simulink model "gimbal_kinematics_model_mpc_v2_19012020"  (R2018b)
settings: Solver=FixedStepAuto  StartTime=0.0  StopTime=10  FixedStep=0.001  MaxStep=0.001  RelTol=1e-3
libraries: robotcorelib x5, mpclib x1
settings Model: Creator=Paweł Tymiński  LastModifiedBy=Paweł Tymiński

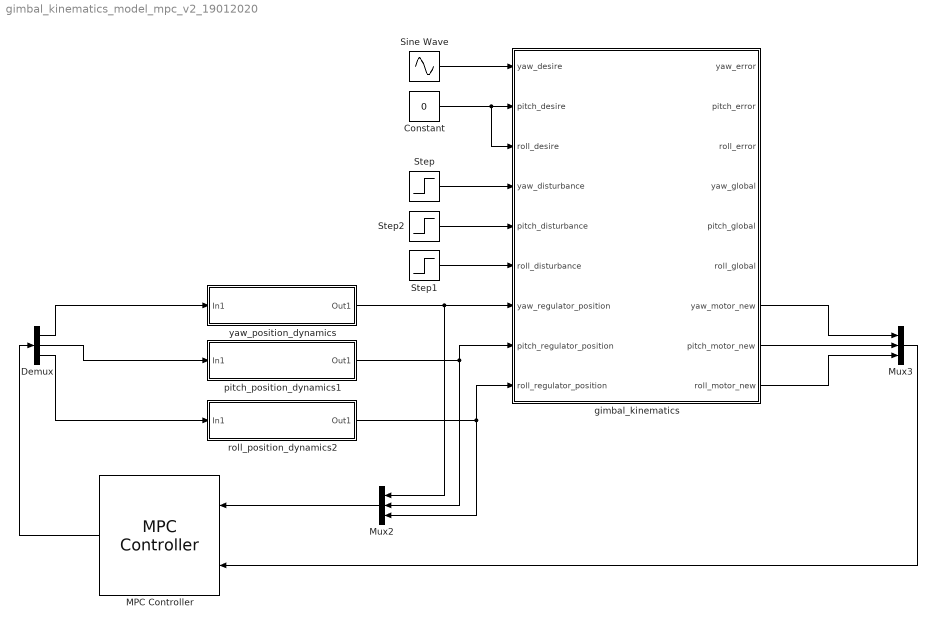
== system gimbal_kinematics_model_mpc_v2_19012020 ==
  Constant : Constant  Value=0
  Demux : Demux  Outputs=3
  MPC Controller : mpclib/MPC Controller  SCDEnableBlockLinearizationSpecification=on  is_multiple=0  enable_value=0  return_u0=off  updateMPCinCallerWorkspace=on  md_inport=off  mv_inport=off  return_cost=off  return_mvseq=off  return_qpstatus=off  return_xseq=off  return_state=off  return_ovseq=off  state_inport=off  umin_inport=off  umax_inport=off  ymin_inport=off  ymax_inport=off  cc_inport=off  ywt_inport=off  uwt_inport=off  duwt_inport=off  rhoeps_inport=off  uref_inport=off  n_ts=0.001  n_p=10  n_mv=3  n_md=0  n_ud=0  n_mo=3  n_uo=0  BlockDataType=double  SampleTimeInherited=off  switch_inport=off
  Mux2 : Mux  Inputs=3
  Mux3 : Mux  Inputs=3
  Sine Wave : Sin  SampleTime=0
  Step : Step  Time=2  After=-0.5  SampleTime=0
  Step1 : Step  Time=2  After=-1  SampleTime=0
  Step2 : Step  Time=5  After=0.5  SampleTime=0
  gimbal_kinematics : Subsystem
  pitch_position_dynamics1 : Subsystem
  roll_position_dynamics2 : Subsystem
  yaw_position_dynamics : Subsystem
  wires:
  pitch_position_dynamics1/1(Out1) -> gimbal_kinematics/8(pitch_regulator_position), Mux2/2
  roll_position_dynamics2/1(Out1) -> gimbal_kinematics/9(roll_regulator_position), Mux2/3
  yaw_position_dynamics/1(Out1) -> Mux2/1, gimbal_kinematics/7(yaw_regulator_position)
  Constant/1 -> gimbal_kinematics/3(roll_desire), gimbal_kinematics/2(pitch_desire)
  Demux/3 -> roll_position_dynamics2/1(In1)
  Demux/2 -> pitch_position_dynamics1/1(In1)
  Step/1 -> gimbal_kinematics/4(yaw_disturbance)
  Step1/1 -> gimbal_kinematics/6(roll_disturbance)
  Demux/1 -> yaw_position_dynamics/1(In1)
  Sine Wave/1 -> gimbal_kinematics/1(yaw_desire)
  Step2/1 -> gimbal_kinematics/5(pitch_disturbance)
  Mux2/1 -> MPC Controller/1
  gimbal_kinematics/8(pitch_motor_new) -> Mux3/2
  gimbal_kinematics/7(yaw_motor_new) -> Mux3/1
  gimbal_kinematics/9(roll_motor_new) -> Mux3/3
  Mux3/1 -> MPC Controller/2
  MPC Controller/1 -> Demux/1

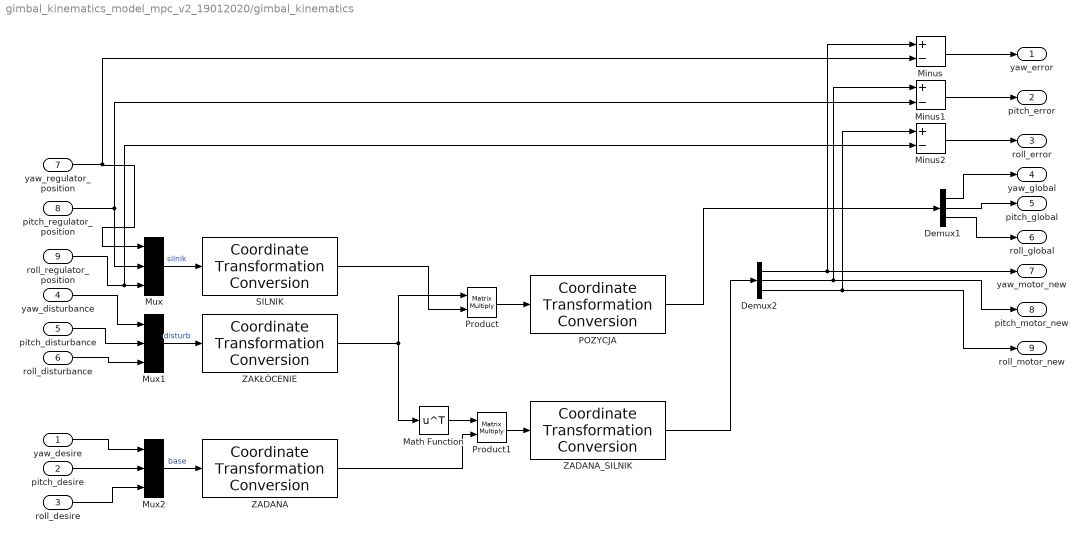
== system gimbal_kinematics_model_mpc_v2_19012020/gimbal_kinematics ==
  yaw_desire : Inport
  pitch_desire : Inport  Port=2
  roll_desire : Inport  Port=3
  yaw_disturbance : Inport  Port=4
  pitch_disturbance : Inport  Port=5
  roll_disturbance : Inport  Port=6
  yaw_regulator_position : Inport  Port=7
  pitch_regulator_position : Inport  Port=8
  roll_regulator_position : Inport  Port=9
  Demux1 : Demux  Outputs=3
  Demux2 : Demux  Outputs=3
  Math Function : Math  Operator=transpose  SaturateOnIntegerOverflow=on
  Minus : Sum  Inputs=+-
  Minus1 : Sum  Inputs=+-
  Minus2 : Sum  Inputs=+-
  Mux : Mux  Inputs=3
  Mux1 : Mux  Inputs=3
  Mux2 : Mux  Inputs=3
  POZYCJA : robotcorelib/Coordinate Transformation Conversion  InputRepresentation=Rotation Matrix  InputEulerSequence=ZYX  ShowTrVecInputPort=on  OutputRepresentation=Euler Angles  OutputEulerSequence=ZYX  ShowTrVecOutputPort=on  SimulateUsing=Interpreted execution
      settings: SourceProductBaseCode=RO
  Product : Product  Multiplication=Matrix(*)
  Product1 : Product  Multiplication=Matrix(*)
  SILNIK : robotcorelib/Coordinate Transformation Conversion  InputRepresentation=Euler Angles  InputEulerSequence=ZYX  ShowTrVecInputPort=on  OutputRepresentation=Rotation Matrix  OutputEulerSequence=ZYX  ShowTrVecOutputPort=on  SimulateUsing=Interpreted execution
      settings: SourceProductBaseCode=RO
  ZADANA : robotcorelib/Coordinate Transformation Conversion  InputRepresentation=Euler Angles  InputEulerSequence=ZYX  ShowTrVecInputPort=on  OutputRepresentation=Rotation Matrix  OutputEulerSequence=ZYX  ShowTrVecOutputPort=on  SimulateUsing=Interpreted execution
      settings: SourceProductBaseCode=RO
  ZADANA_SILNIK : robotcorelib/Coordinate Transformation Conversion  InputRepresentation=Rotation Matrix  InputEulerSequence=ZYX  ShowTrVecInputPort=on  OutputRepresentation=Euler Angles  OutputEulerSequence=ZYX  ShowTrVecOutputPort=on  SimulateUsing=Interpreted execution
      settings: SourceProductBaseCode=RO
  ZAKŁÓCENIE : robotcorelib/Coordinate Transformation Conversion  InputRepresentation=Euler Angles  InputEulerSequence=ZYX  ShowTrVecInputPort=on  OutputRepresentation=Rotation Matrix  OutputEulerSequence=ZYX  ShowTrVecOutputPort=on  SimulateUsing=Interpreted execution
      settings: SourceProductBaseCode=RO
  yaw_error : Outport
  pitch_error : Outport  Port=2
  roll_error : Outport  Port=3
  yaw_global : Outport  Port=4
  pitch_global : Outport  Port=5
  roll_global : Outport  Port=6
  yaw_motor_new : Outport  Port=7
  pitch_motor_new : Outport  Port=8
  roll_motor_new : Outport  Port=9
  wires:
  ZADANA_SILNIK/1 -> Demux2/1
  ZADANA/1 -> Product1/2
  Product/1 -> POZYCJA/1
  Mux1/1 -> ZAKŁÓCENIE/1  "disturb"
  SILNIK/1 -> Product/2
  Math Function/1 -> Product1/1
  Product1/1 -> ZADANA_SILNIK/1
  Mux/1 -> SILNIK/1  "silnik"
  Mux2/1 -> ZADANA/1  "base"
  ZAKŁÓCENIE/1 -> Math Function/1, Product/1
  pitch_desire/1 -> Mux2/2
  yaw_desire/1 -> Mux2/1
  roll_desire/1 -> Mux2/3
  yaw_disturbance/1 -> Mux1/1
  pitch_disturbance/1 -> Mux1/2
  roll_disturbance/1 -> Mux1/3
  roll_regulator_position/1 -> Mux/3, Minus2/2
  pitch_regulator_position/1 -> Mux/2, Minus1/2
  yaw_regulator_position/1 -> Mux/1, Minus/2
  Demux1/2 -> pitch_global/1
  Demux1/1 -> yaw_global/1
  Demux1/3 -> roll_global/1
  Demux2/1 -> Minus/1, yaw_motor_new/1
  Demux2/2 -> Minus1/1, pitch_motor_new/1
  Demux2/3 -> Minus2/1, roll_motor_new/1
  Minus/1 -> yaw_error/1
  POZYCJA/1 -> Demux1/1
  Minus1/1 -> pitch_error/1
  Minus2/1 -> roll_error/1

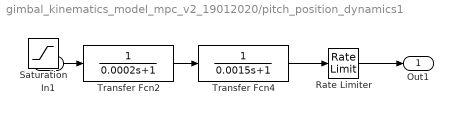
== system gimbal_kinematics_model_mpc_v2_19012020/pitch_position_dynamics1 ==
  In1 : Inport
  Rate Limiter : RateLimiter  RisingSlewLimit=18.5  FallingSlewLimit=-18.5  SampleTimeMode=inherited
  Saturation : Saturate  UpperLimit=58.5  LowerLimit=-58.5
  Transfer Fcn2 : TransferFcn  Denominator=[0.0002 1]
  Transfer Fcn4 : TransferFcn  Denominator=[0.0015 1]
  Out1 : Outport
  wires:
  Transfer Fcn2/1 -> Transfer Fcn4/1
  In1/1 -> Transfer Fcn2/1
  Transfer Fcn4/1 -> Rate Limiter/1
  Rate Limiter/1 -> Out1/1

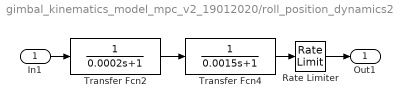
== system gimbal_kinematics_model_mpc_v2_19012020/roll_position_dynamics2 ==
  In1 : Inport
  Rate Limiter : RateLimiter  RisingSlewLimit=18.5  FallingSlewLimit=-18.5  SampleTimeMode=inherited
  Transfer Fcn2 : TransferFcn  Denominator=[0.0002 1]
  Transfer Fcn4 : TransferFcn  Denominator=[0.0015 1]
  Out1 : Outport
  wires:
  Transfer Fcn2/1 -> Transfer Fcn4/1
  In1/1 -> Transfer Fcn2/1
  Transfer Fcn4/1 -> Rate Limiter/1
  Rate Limiter/1 -> Out1/1

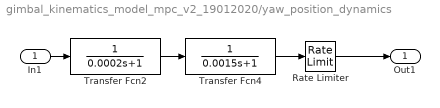
== system gimbal_kinematics_model_mpc_v2_19012020/yaw_position_dynamics ==
  In1 : Inport
  Rate Limiter : RateLimiter  RisingSlewLimit=18.5  FallingSlewLimit=-18.5  SampleTimeMode=inherited
  Transfer Fcn2 : TransferFcn  Denominator=[0.0002 1]
  Transfer Fcn4 : TransferFcn  Denominator=[0.0015 1]
  Out1 : Outport
  wires:
  Transfer Fcn2/1 -> Transfer Fcn4/1
  In1/1 -> Transfer Fcn2/1
  Transfer Fcn4/1 -> Rate Limiter/1
  Rate Limiter/1 -> Out1/1
